simulink subsystem "Averaging"  (R2024b)
settings: Solver=VariableStepAuto  StartTime=0.0  StopTime=10.0  RelTol=1e-3
libraries: simulink x1
settings Model: Creator=phippold  LastModifiedBy=phippold

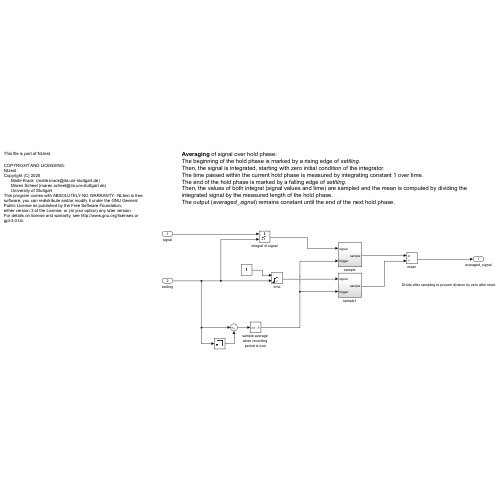
[thumbnail: Simulink's stored preview of the top-level diagram]
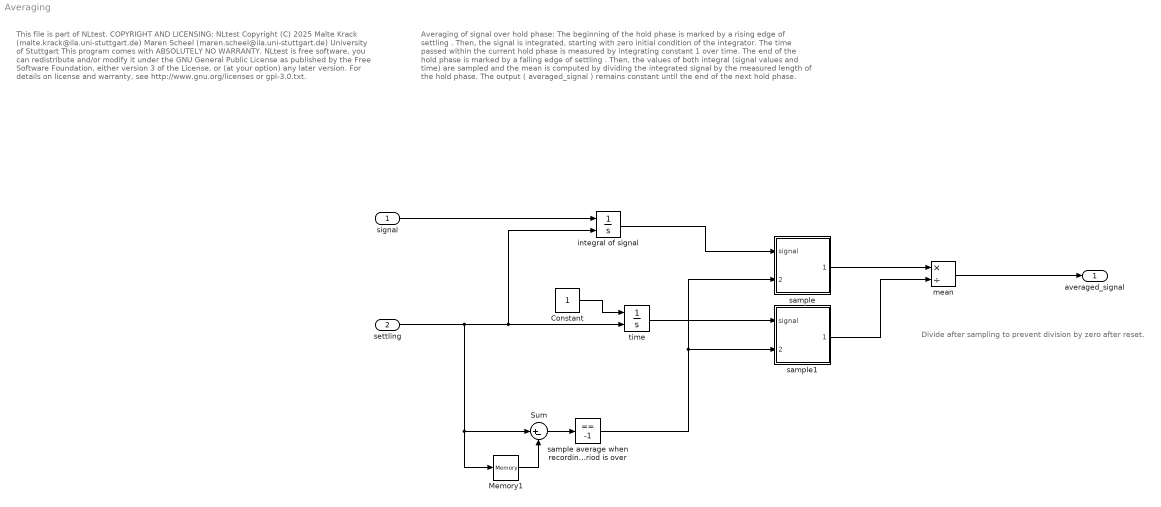
== system Averaging ==
  note: Divide after sampling to prevent division by zero after reset.
  note: Averaging of signal over hold phase:
      | The beginning of the hold phase is marked by a rising edge of settling .
      | Then, the signal is integrated, starting with zero initial condition of the integrator.
      | The time passed within the current hold phase is measured by integrating constant 1 over time.
      | The end of the hold phase is marked by a falling edge of settling .
      | Then, the values of both integral (signal values and time) are sampled and the mean is computed by dividing the integrated signal by the measured length of the hold phase.
      | The output ( averaged_signal ) remains constant until the end of the next hold phase.
  note: This file is part of NLtest.
      |
      | COPYRIGHT AND LICENSING:
      | NLtest
      | Copyright (C) 2025
      | Malte Krack (malte.krack@ila.uni-stuttgart.de)
      | Maren Scheel (maren.scheel@ila.uni-stuttgart.de)
      | University of Stuttgart
      | This program comes with ABSOLUTELY NO WARRANTY. NLtest is free software, you can redistribute and/or modify it under the GNU General Public License as published by the Free Software Foundation,
      | either version 3 of the License, or (at your option) any later version.
      | For details on license and warranty, see http://www.gnu.org/licenses or gpl-3.0.txt.
  signal : Inport
  settling : Inport  Port=2
  Constant : Constant
  Memory1 : Memory
  Sum : Sum  Inputs=|+-  OutDataTypeStr=double
  integral of signal : Integrator  ExternalReset=rising
  mean : Product  Inputs=*/
  sample : Subsystem
  sample average when recording period is over : simulink/Logic and Bit Operations/Compare To Constant  relop===  const=-1  OutDataTypeStr=boolean
  sample1 : Subsystem
  time : Integrator  ExternalReset=rising
  averaged_signal : Outport
  wires:
  signal/1 -> integral of signal/1
  sample1/1(sample) -> mean/2
  sample/1(sample) -> mean/1
  sample average when recording period is over/1 -> sample1/2(trigger), sample/2(trigger)
  Memory1/1 -> Sum/2
  Sum/1 -> sample average when recording period is over/1
  settling/1 -> time/2, integral of signal/2, Sum/1, Memory1/1
  mean/1 -> averaged_signal/1
  time/1 -> sample1/1(signal)
  integral of signal/1 -> sample/1(signal)
  Constant/1 -> time/1

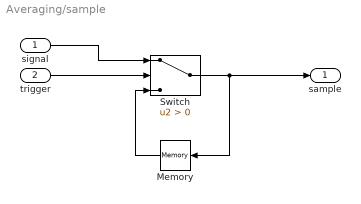
== system Averaging/sample ==
  signal : Inport
  trigger : Inport  Port=2
  Memory : Memory  InitialCondition=nan
  Switch : Switch  Criteria=u2 > Threshold  SaturateOnIntegerOverflow=off  InputSameDT=off
  sample : Outport
  wires:
  trigger/1 -> Switch/2
  Switch/1 -> Memory/1, sample/1
  Memory/1 -> Switch/3
  signal/1 -> Switch/1

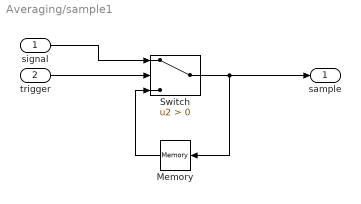
== system Averaging/sample1 ==
  signal : Inport
  trigger : Inport  Port=2
  Memory : Memory  InitialCondition=1
  Switch : Switch  Criteria=u2 > Threshold  SaturateOnIntegerOverflow=off  InputSameDT=off
  sample : Outport
  wires:
  trigger/1 -> Switch/2
  Switch/1 -> Memory/1, sample/1
  Memory/1 -> Switch/3
  signal/1 -> Switch/1
